simulink model "WalkingCaneSystem"  (R2023b)
settings: Solver=VariableStepAuto  StartTime=0.0  StopTime=inf  FixedStep=0.01  RelTol=1e-3  EnableMultiTasking=on
model workspace (MAT data in the model file):
  SL_ROS_VariableLengthArrays_MaxSizes.CommonInfo.ArrayTruncateAction = 'EmitWarning'
  SL_ROS_VariableLengthArrays_MaxSizes.MsgTypeMap = containers.Map
  SL_ROS_VariableLengthArrays_MaxSizes.MsgTypeMap.serialization.keys = {'sensor_msgs/LaserScan'}
  SL_ROS_VariableLengthArrays_MaxSizes.MsgTypeMap.serialization.values{1}(1).PropertyName = 'Intensities'
  SL_ROS_VariableLengthArrays_MaxSizes.MsgTypeMap.serialization.values{1}(1).DataType = 'single'
  SL_ROS_VariableLengthArrays_MaxSizes.MsgTypeMap.serialization.values{1}(1).MaxLength = 360
  SL_ROS_VariableLengthArrays_MaxSizes.MsgTypeMap.serialization.values{1}(2).PropertyName = 'Ranges'
  SL_ROS_VariableLengthArrays_MaxSizes.MsgTypeMap.serialization.values{1}(2).DataType = 'single'
  SL_ROS_VariableLengthArrays_MaxSizes.MsgTypeMap.serialization.values{1}(2).MaxLength = 360
  SL_ROS_VariableLengthArrays_MaxSizes.MsgTypeMap.serialization.uniformity = 0
  SL_ROS_VariableLengthArrays_MaxSizes.MsgTypeMap.serialization.keyType = 'char'
  SL_ROS_VariableLengthArrays_MaxSizes.MsgTypeMap.serialization.valueType = 'any'
values from neighbouring files (symbols this model uses):
  scan = lidarScan(scanMsg)    [WalkingCaneWanderer.m]
undefined symbols (not defined in the file or in its folder): Angular, Linear
libraries: robotlib x4, robotalgslib x2
settings Model: Creator=The MathWorks, Inc.  LastModifiedBy=needs
settings SolverCC: AlgebraicLoopSolver=TrustRegion
settings DataIOCC: ReturnWorkspaceOutputs=off
settings DebuggingCC: UnconnectedInputMsg=warning  UnconnectedOutputMsg=warning  UnconnectedLineMsg=warning  ArithmeticOperatorsInVariantConditions=warning
settings ModelReferenceCC: EnableRefExpFcnMdlSchedulingChecks=on
settings SFSimCC: SimUseLocalCustomCode=off  CustomCodeUndefinedFunction=UseInterfaceOnly
settings RTWCC: RTWUseLocalCustomCode=off
settings CodeAppCC: StateflowObjectComments=on
settings GRTTargetCC: TargetLangStandard=C89/C90 (ANSI)
settings ConfigComp: CovMetricSettings=dsw  CovSaveCumulativeToWorkspaceVar=on  CovSaveSingleToWorkspaceVar=on  CovExternalEMLEnable=off

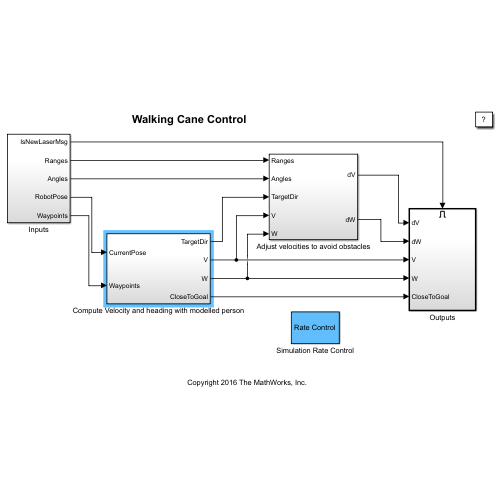
[thumbnail: Simulink's stored preview of the top-level diagram]
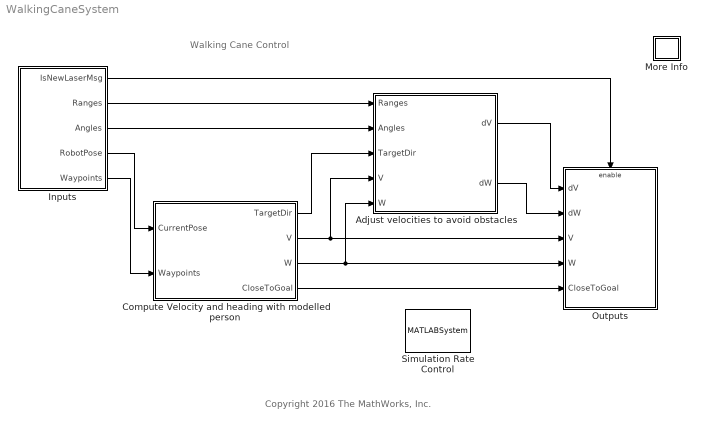
== system WalkingCaneSystem ==
  note: Walking Cane Control
  note: Copyright 2016 The MathWorks, Inc.
  Adjust velocities to avoid obstacles : Subsystem
  Compute Velocity and heading with modelled person : Subsystem
  Inputs : Subsystem
  More Info : Subsystem
      settings: OpenFcn=showdemo(bdroot(gcb))
      mask Display: disp('?')
  Outputs : Subsystem
  Simulation Rate Control : MATLABSystem  System=ExampleHelperSimulationRateControl  SampleTime=0.02
      mask Type: ExampleHelperSimulationRateControl
      mask Display: disp('Rate Control');
  wires:
  Compute Velocity and heading with modelled person/2(V) -> Outputs/3(V), Adjust velocities to avoid obstacles/4(V)
  Compute Velocity and heading with modelled person/1(TargetDir) -> Adjust velocities to avoid obstacles/3(TargetDir)
  Inputs/2(Ranges) -> Adjust velocities to avoid obstacles/1(Ranges)
  Inputs/3(Angles) -> Adjust velocities to avoid obstacles/2(Angles)
  Inputs/1(IsNewLaserMsg) -> Outputs/Enable
  Inputs/4(RobotPose) -> Compute Velocity and heading with modelled person/1(CurrentPose)
  Inputs/5(Waypoints) -> Compute Velocity and heading with modelled person/2(Waypoints)
  Compute Velocity and heading with modelled person/3(W) -> Outputs/4(W), Adjust velocities to avoid obstacles/5(W)
  Adjust velocities to avoid obstacles/1(dV) -> Outputs/1(dV)
  Adjust velocities to avoid obstacles/2(dW) -> Outputs/2(dW)
  Compute Velocity and heading with modelled person/4(CloseToGoal) -> Outputs/5(CloseToGoal)

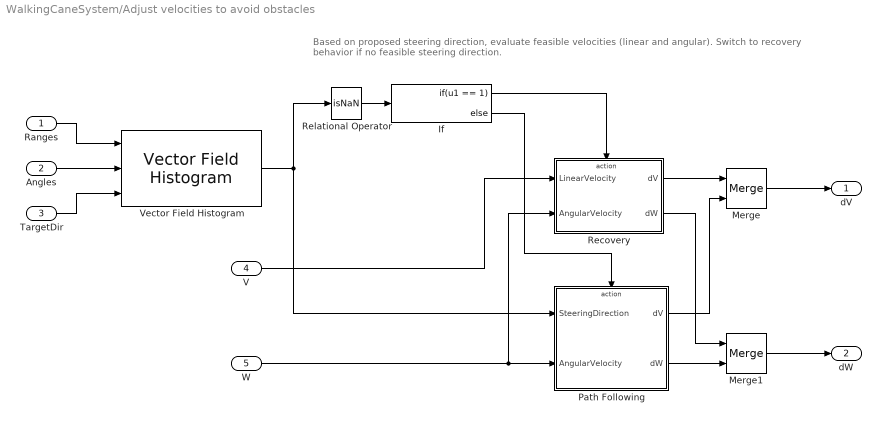
== system WalkingCaneSystem/Adjust velocities to avoid obstacles ==
  note: Based on proposed steering direction, evaluate feasible velocities (linear and angular).
      | 				Switch to recovery behavior if no feasible steering direction.
  Ranges : Inport
  Angles : Inport  Port=2
  TargetDir : Inport  Port=3
  V : Inport  Port=4
  W : Inport  Port=5
  If : If  IfExpression=u1 == 1
  Merge : Merge
  Merge1 : Merge
  Path Following : Subsystem  TreatAsAtomicUnit=on
  Recovery : Subsystem  TreatAsAtomicUnit=on
  Relational Operator : RelationalOperator  Operator=isNaN  OutDataTypeStr=boolean  RndMeth=Simplest  InputSameDT=off
  Vector Field Histogram : robotalgslib/Vector Field Histogram  NumAngularSectors=180  DistanceLimits=[ 0.05, 3 ]  HistogramThresholds=[ 3, 8 ]  RobotRadius=0.2  SafetyDistance=0.2  MinTurningRadius=0.2  SimulateUsing=Code generation  TargetDirectionWeight=5  CurrentDirectionWeight=2  PreviousDirectionWeight=2
  dV : Outport  VectorParamsAs1DForOutWhenUnconnected=off
  dW : Outport  Port=2  VectorParamsAs1DForOutWhenUnconnected=off
  wires:
  Merge1/1 -> dW/1
  V/1 -> Recovery/1(LinearVelocity)
  Vector Field Histogram/1 -> Relational Operator/1, Path Following/1(SteeringDirection)
  W/1 -> Recovery/2(AngularVelocity), Path Following/2(AngularVelocity)
  Relational Operator/1 -> If/1
  Angles/1 -> Vector Field Histogram/2
  Merge/1 -> dV/1
  TargetDir/1 -> Vector Field Histogram/3
  Ranges/1 -> Vector Field Histogram/1
  If/1 -> Recovery/Action
  If/2 -> Path Following/Action
  Recovery/2(dW) -> Merge1/1
  Path Following/2(dW) -> Merge1/2
  Recovery/1(dV) -> Merge/1
  Path Following/1(dV) -> Merge/2

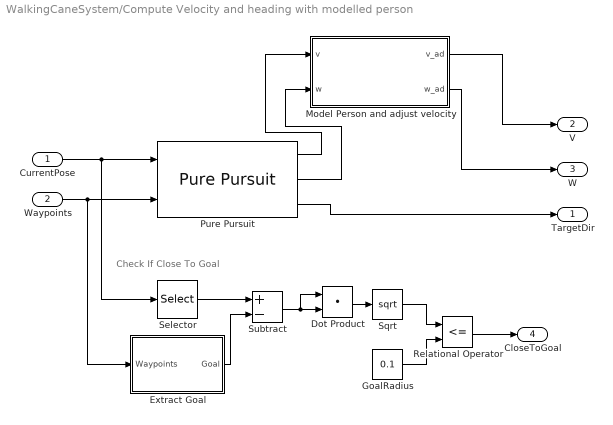
== system WalkingCaneSystem/Compute Velocity and heading with modelled person ==
  note: Check If Close To Goal
  CurrentPose : Inport
  Waypoints : Inport  Port=2
  " Extract Goal" : MATLAB Function  TreatAsAtomicUnit=on
  Dot Product : DotProduct  OutDataTypeStr=Inherit: Inherit via internal rule
  GoalRadius : Constant  Value=0.1
  Model Person and adjust velocity : MATLAB Function  TreatAsAtomicUnit=on
  Pure Pursuit : robotalgslib/Pure Pursuit  DesiredLinearVelocity=0.3  MaxAngularVelocity=1.0  LookaheadDistance=2.0  TargetDirPort=on  SimulateUsing=Code generation
  Relational Operator : RelationalOperator  Operator=<=  OutDataTypeStr=boolean  RndMeth=Simplest  InputSameDT=off
  Selector : Selector  InputPortWidth=3  IndexOptions=Index vector (dialog)  Indices=[1 2]  OutputSizes=1
  Sqrt : Sqrt
  Subtract : Sum  Inputs=+-
  TargetDir : Outport  VectorParamsAs1DForOutWhenUnconnected=off
  V : Outport  Port=2  VectorParamsAs1DForOutWhenUnconnected=off
  W : Outport  Port=3  VectorParamsAs1DForOutWhenUnconnected=off
  CloseToGoal : Outport  Port=4  VectorParamsAs1DForOutWhenUnconnected=off
  wires:
  Pure Pursuit/3 -> TargetDir/1
  Pure Pursuit/2 -> Model Person and adjust velocity/2(w)
  Pure Pursuit/1 -> Model Person and adjust velocity/1(v)
  " Extract Goal"/1(Goal) -> Subtract/2
  Waypoints/1 -> " Extract Goal"/1(Waypoints), Pure Pursuit/2
  CurrentPose/1 -> Selector/1, Pure Pursuit/1
  Relational Operator/1 -> CloseToGoal/1
  GoalRadius/1 -> Relational Operator/2
  Selector/1 -> Subtract/1
  Dot Product/1 -> Sqrt/1
  Sqrt/1 -> Relational Operator/1
  Subtract/1 -> Dot Product/1, Dot Product/2
  Model Person and adjust velocity/1(v_ad) -> V/1
  Model Person and adjust velocity/2(w_ad) -> W/1

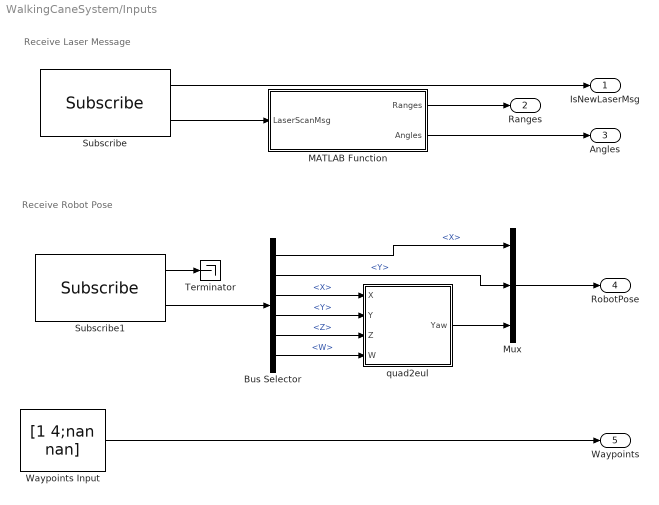
== system WalkingCaneSystem/Inputs ==
  note: Receive Robot Pose
  note: Receive Laser Message
  Bus Selector : BusSelector  OutputSignals=Pose.Pose.Position.X,Pose.Pose.Position.Y,Pose.Pose.Orientation.X,Pose.Pose.Orientation.Y,Pose.Pose.Orientation.Z,Pose.Pose.Orientation.W
  MATLAB Function : MATLAB Function  TreatAsAtomicUnit=on
  Mux : Mux  Inputs=3
  Subscribe : robotlib/Subscribe  topicSource=Select from ROS network  topic=/scan  messageType=sensor_msgs/LaserScan  SampleTime=-1  legacyBusStruct=off  messageQueueLength=1
  Subscribe1 : robotlib/Subscribe  topicSource=Select from ROS network  topic=/odom  messageType=nav_msgs/Odometry  SampleTime=-1  legacyBusStruct=off  messageQueueLength=1
  Terminator : Terminator
  Waypoints Input : Constant  Value=[1 4;nan nan]  OutDataTypeStr=double
  quad2eul : MATLAB Function  TreatAsAtomicUnit=on
  IsNewLaserMsg : Outport  VectorParamsAs1DForOutWhenUnconnected=off
  Ranges : Outport  Port=2  VectorParamsAs1DForOutWhenUnconnected=off
  Angles : Outport  Port=3  VectorParamsAs1DForOutWhenUnconnected=off
  RobotPose : Outport  Port=4  VectorParamsAs1DForOutWhenUnconnected=off
  Waypoints : Outport  Port=5  VectorParamsAs1DForOutWhenUnconnected=off
  wires:
  Waypoints Input/1 -> Waypoints/1
  Subscribe/2 -> MATLAB Function/1(LaserScanMsg)
  quad2eul/1(Yaw) -> Mux/3
  Subscribe1/2 -> Bus Selector/1
  Bus Selector/3 -> quad2eul/1(X)  "<X>"
  Subscribe1/1 -> Terminator/1
  Bus Selector/2 -> Mux/2  "<Y>"
  Bus Selector/5 -> quad2eul/3(Z)  "<Z>"
  Bus Selector/4 -> quad2eul/2(Y)  "<Y>"
  Bus Selector/1 -> Mux/1  "<X>"
  Bus Selector/6 -> quad2eul/4(W)  "<W>"
  MATLAB Function/1(Ranges) -> Ranges/1
  MATLAB Function/2(Angles) -> Angles/1
  Subscribe/1 -> IsNewLaserMsg/1
  Mux/1 -> RobotPose/1

== system WalkingCaneSystem/More Info ==

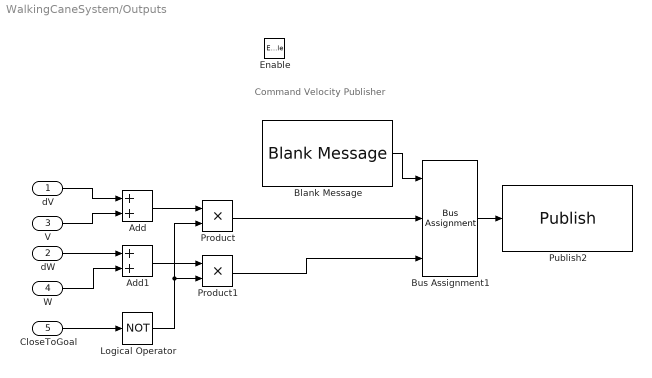
== system WalkingCaneSystem/Outputs ==
  note: Command Velocity Publisher
  dV : Inport
  dW : Inport  Port=2
  V : Inport  Port=3
  W : Inport  Port=4
  CloseToGoal : Inport  Port=5
  Enable : EnablePort
  Add : Sum
  Add1 : Sum
  Blank Message : robotlib/Blank Message  messageClass=Message  entityType=geometry_msgs/Twist  messageType=geometry_msgs/Twist  SampleTime=inf  legacyBusStruct=off
  Bus Assignment1 : BusAssignment  DialogController=Simulink.DDGSource_BusAssignment  AssignedSignals=Linear.X,Angular.Z
  Logical Operator : Logic  Operator=NOT  AllPortsSameDT=off  OutDataTypeStr=boolean
  Product : Product
  Product1 : Product
  Publish2 : robotlib/Publish  topicSource=Select from ROS network  topic=/cmd_vel  messageType=geometry_msgs/Twist  legacyBusStruct=off  messageQueueLength=105
  wires:
  V/1 -> Add/2
  W/1 -> Add1/2
  dV/1 -> Add/1
  dW/1 -> Add1/1
  CloseToGoal/1 -> Logical Operator/1
  Add/1 -> Product/1
  Add1/1 -> Product1/1
  Product1/1 -> Bus Assignment1/3
  Product/1 -> Bus Assignment1/2
  Blank Message/1 -> Bus Assignment1/1
  Bus Assignment1/1 -> Publish2/1
  Logical Operator/1 -> Product1/2, Product/2

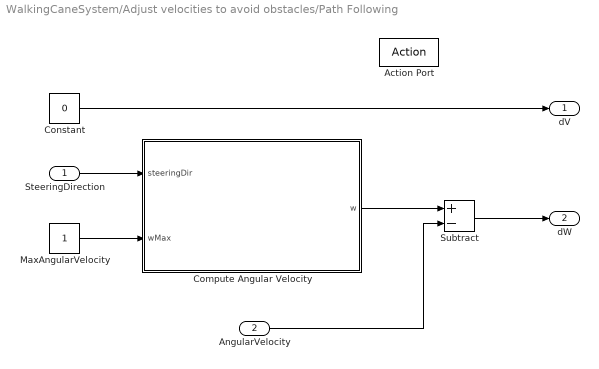
== system WalkingCaneSystem/Adjust velocities to avoid obstacles/Path Following ==
  SteeringDirection : Inport
  AngularVelocity : Inport  Port=2
  Action Port : ActionPort  ActionPortLabel=else
  Compute Angular Velocity : MATLAB Function  TreatAsAtomicUnit=on
  Constant : Constant  Value=0
  MaxAngularVelocity : Constant
  Subtract : Sum  Inputs=+-
  dV : Outport  VectorParamsAs1DForOutWhenUnconnected=off
  dW : Outport  Port=2  VectorParamsAs1DForOutWhenUnconnected=off
  wires:
  Constant/1 -> dV/1
  MaxAngularVelocity/1 -> Compute Angular Velocity/2(wMax)
  SteeringDirection/1 -> Compute Angular Velocity/1(steeringDir)
  Subtract/1 -> dW/1
  Compute Angular Velocity/1(w) -> Subtract/1
  AngularVelocity/1 -> Subtract/2

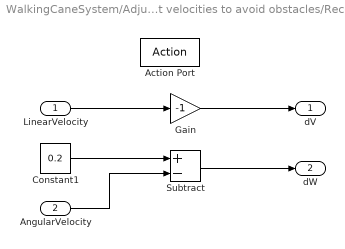
== system WalkingCaneSystem/Adjust velocities to avoid obstacles/Recovery ==
  LinearVelocity : Inport
  AngularVelocity : Inport  Port=2
  Action Port : ActionPort  ActionPortLabel=if(u1 == 1)
  Constant1 : Constant  Value=0.2
  Gain : Gain  Gain=-1
  Subtract : Sum  Inputs=+-
  dV : Outport  VectorParamsAs1DForOutWhenUnconnected=off
  dW : Outport  Port=2  VectorParamsAs1DForOutWhenUnconnected=off
  wires:
  LinearVelocity/1 -> Gain/1
  Gain/1 -> dV/1
  Constant1/1 -> Subtract/1
  AngularVelocity/1 -> Subtract/2
  Subtract/1 -> dW/1

== matlab function WalkingCaneSystem/Inputs/quad2eul ==
  data: X input; Yaw output; Y input; Z input; W input
function Yaw = quat2eulBlk(X, Y, Z, W)
%#codegen

eularAngles = quat2eul([W, X, Y, Z]);
Yaw = eularAngles(1);

== matlab function WalkingCaneSystem/Compute Velocity and heading with modelled person/Model Person and adjust velocity ==
  data: v input; v_ad output; w input; w_ad output
function [v_ad, w_ad] = adjust_velocity(v,w)
w
v_ad = v;
w_ad = w;

    % Constants for PID control
    Kp_v = 1;   % Proportional gain for linear velocity
    Kd_v = 0.2; % Derivative gain for linear velocity

    Kp_w = 1;   % Proportional gain for angular velocity
    Kd_w = 0.2; % Derivative gain for angular velocity

    % Generate random values for v_person and w_person between a and b
    v_person = 0.1 + (0.5 - 0.1) * rand();
    w_person = 0.1 + (0.5 - 0.1) * rand();

    % PID control for linear velocity
    error_v = v_person - v;
    derivative_v = 0;

    % Update PID terms

    derivative_v = error_v;

    % Calculate control signal for linear velocity
    control_signal_v = Kp_v * error_v  + Kd_v * derivative_v;

    % PID control for angular velocity
    error_w = w_person - w;
    derivative_w = 0;

    % Update PID terms
    derivative_w = error_w;

    % Calculate control signal for angular velocity
    control_signal_w = Kp_w * error_w  + Kd_w * derivative_w;

    % Adjust linear and angular velocity based on control signals
    v_adjusted = v + control_signal_v;
    w_adjusted = w + control_signal_w;

    % Display results

end

== matlab function WalkingCaneSystem/Inputs/MATLAB Function ==
  data: LaserScanMsg input; Ranges output; Angles output
function [Ranges, Angles] = ExtractRangeData(LaserScanMsg)
%#codegen

% Extract Range information
Ranges = double(LaserScanMsg.Ranges);

% Construct Angles vector using AngleMin and AngleIncrement from sensor
% reading.
angMin = double(LaserScanMsg.AngleMin);
angIncrement = double(LaserScanMsg.AngleIncrement);

numReadings = numel(Ranges);
rawAngles = angMin + (0:numReadings-1)' * angIncrement;

% Wrap the angles to the (-pi,pi] interval.
Angles = robotics.internal.wrapToPi(double(rawAngles));

== matlab function WalkingCaneSystem/Compute Velocity and heading with modelled person/ Extract Goal ==
  data: Waypoints input; Goal output
function Goal = extractGoal(Waypoints)
%#codegen
b = isnan(Waypoints);
[rows,~] = find(b);
ridx = setdiff(1:size(Waypoints,1), sort(rows));
Goal = [Waypoints(ridx(end), 1) Waypoints(ridx(end), 2)];

== matlab function WalkingCaneSystem/Adjust velocities to avoid obstacles/Path Following/Compute Angular Velocity ==
  data: steeringDir input; w output; wMax input
function w = exampleHelperComputeAngularVelocity(steeringDir, wMax)
%EXAMPLEHELPERCOMPUTEANGULARVELOCITY Compute angular velocity
%   W = exampleHelperComputeAngularVelocity(STEERINGDIR)
%   returns the angular velocity W for a differential drive robot in radians
%   per second for a given steering direction STEERINGDIR in the robot's
%   coordinate frame in radians.
%
%   W = exampleHelperComputeAngularVelocity(STEERINGDIR, WMAX)
%   returns the angular velocity W for a differential drive robot in radians
%   per second for a given steering direction STEERINGDIR in the robot's
%   coordinate frame in radians and maximum angular velocity WMAX in
%   radians per second. The output angular velocity is saturated based on
%   the WMAX.
%
%   Example:
%       
%       w = exampleHelperComputeAngularVelocity(0.2, 1);

% Copyright 2015 The MathWorks, Inc.

%#codegen
%#ok<*EMCA>

% Allow variable input arguments
if nargin == 1   
    wMax = inf;
end

validateattributes(steeringDir, {'double'},{'real'},...
    'exampleHelperComputeAngularVelocity', 'STEERINGDIR', 1);
validateattributes(wMax, {'double'},{'real', 'positive'},...
    'exampleHelperComputeAngularVelocity', 'WMAX', 2);

% Computing in robot's coordinate frame
curPose = [0 0 0];

% The following computation is similar to robotics.PurePursuit
lookaheadPoint = [cos(steeringDir), sin(steeringDir)];
slope = atan2((lookaheadPoint(2) - curPose(2)), ...
    (lookaheadPoint(1) - curPose(1)));
alpha = angdiff(curPose(3), slope);

% Angular velocity command for a differential drive robot is
% equal to the desired curvature to be followed by the robot.

w = (2*sin(alpha));

% Pick a constant rotation when robot is facing in the opposite
% direction of the path
if abs(abs(alpha) - pi) < 1e-12
    w = sign(w)*1;
end

if abs(w) > wMax
    w = sign(w)*wMax;
end

end
